simulink model "IEEE_39_case7"  (R2024b)
settings: Solver=ode3  StartTime=0  StopTime=40  FixedStep=Ts  MaxStep=1/60  RelTol=1e-3  AbsTol=1e-3  EnableMultiTasking=on
values from neighbouring files (symbols this model uses):
  c_f = c_f*Cb    [fun00_GFL_pu_2_normial.m]    (also in fun00_GFM_pu_2_normial.m)
  Dt = 0    [s02_case1.m]    (also in s02_case2.m; s03_case3.m; s03_case4.m; s03_case5.m)
  dw0_sm = 0    [s02_case1.m]    (also in s02_case2.m; s03_case3.m; s03_case4.m; s03_case5.m)
  Emax = 1.3    [s02_case1.m]    (also in s02_case2.m; s03_case3.m; s03_case4.m; s03_case5.m)
  Emin = 0.5    [s02_case1.m]    (also in s02_case2.m; s03_case3.m; s03_case4.m; s03_case5.m)
  Epss = 0.09    [s02_case1.m]    (also in s02_case2.m; s03_case3.m; s03_case4.m; s03_case5.m)
  fb = fn    (= 60)    [s02_case1.m]    (also in s02_case2.m; s03_case3.m; s03_case4.m; s03_case5.m)
  fn_sm = fn*ones(1,10)    [s02_case1.m]    (also in s02_case2.m; s03_case3.m; s03_case4.m; s03_case5.m)
  H_sm = [5,3.03,3.58,2.86,2.6,3.48,2.64,2.43,3.45,4.2]    [s02_case1.m]    (also in s02_case2.m; s03_case3.m; s03_case4.m; s03_case5.m)
  ia0_sm = 0    [s02_case1.m]    (also in s02_case2.m; s03_case3.m; s03_case4.m; s03_case5.m)
  ib0_sm = 0    [s02_case1.m]    (also in s02_case2.m; s03_case3.m; s03_case4.m; s03_case5.m)
  ic0_sm = 0    [s02_case1.m]    (also in s02_case2.m; s03_case3.m; s03_case4.m; s03_case5.m)
  Kd_sm = 0*ones(1,10)    [s02_case1.m]    (also in s02_case2.m; s03_case3.m; s03_case4.m; s03_case5.m)
  Ke = 1000    [s02_case1.m]    (also in s02_case2.m; s03_case3.m; s03_case4.m; s03_case5.m)
  ki_i = ki_i_pu*Vb_p_ph/Ib_p_ph    [fun00_GFL_pu_2_normial.m]    (also in fun00_GFM_pu_2_normial.m)
  ki_p = ki_p_pu/Sb*Ib_p_ph    [fun00_GFL_pu_2_normial.m]
  ki_pll = ki_pll/Vb_p_ph    [fun00_GFL_pu_2_normial.m]
  ki_q = ki_q_pu/Sb*Ib_p_ph    [fun00_GFL_pu_2_normial.m]
  kp_i = kp_i_pu*Vb_p_ph/Ib_p_ph    [fun00_GFL_pu_2_normial.m]    (also in fun00_GFM_pu_2_normial.m)
  kp_p = kp_p_pu/Sb*Ib_p_ph    [fun00_GFL_pu_2_normial.m]
  kp_pll = kp_pll/Vb_p_ph    [fun00_GFL_pu_2_normial.m]
  kp_q = kp_q_pu/Sb*Ib_p_ph    [fun00_GFL_pu_2_normial.m]
  Ks = 1    [s02_case1.m]    (also in s02_case2.m; s03_case3.m; s03_case4.m; s03_case5.m)
  l_f = l_f*Lb    [fun00_GFL_pu_2_normial.m]    (also in fun00_GFM_pu_2_normial.m)
  line = [     1	2	0.0035	0.0411	0.6987	0	100	345 ... (first row only)    [s02_case1.m]    (also in s02_case2.m; s03_case3.m; s03_case4.m; s03_case5.m)
  line_pu = line    [s02_case1.m]    (also in s02_case2.m; s03_case3.m; s03_case4.m; s03_case5.m)
  p = 1    [s02_case1.m]    (also in s02_case2.m; s03_case3.m; s03_case4.m; s03_case5.m)
  pha0_sm = 0    [s02_case1.m]    (also in s02_case2.m; s03_case3.m; s03_case4.m; s03_case5.m)
  phb0_sm = 0    [s02_case1.m]    (also in s02_case2.m; s03_case3.m; s03_case4.m; s03_case5.m)
  phc0_sm = 0    [s02_case1.m]    (also in s02_case2.m; s03_case3.m; s03_case4.m; s03_case5.m)
  Pn_sm = 1000*ones(1,num_gen)    [s02_case1.m]    (also in s02_case2.m; s03_case3.m; s03_case4.m; s03_case5.m)
  Pref_sm = [500 250 600 978 510 650 560 540 830 550]./Pn_sm    [s02_case1.m]    (also in s02_case2.m; s03_case3.m; s03_case4.m; s03_case5.m)
  pset = p_set_pu*Sb    [fun00_GFL_pu_2_normial.m]
  qset = q_set_pu*Sb    [fun00_GFL_pu_2_normial.m]
  R = 0.05    [s02_case1.m]    (also in s02_case2.m; s03_case3.m; s03_case4.m; s03_case5.m)
  r_f = r_f*Zb    [fun00_GFL_pu_2_normial.m]    (also in fun00_GFM_pu_2_normial.m)
  rs = 0.28    [s02_case1.m]    (also in s02_case2.m; s03_case3.m; s03_case4.m; s03_case5.m)
  Sb = 1000*10^6    (= 1000000000)    [s02_case1.m]    (also in s02_case2.m; s03_case3.m; s03_case4.m; s03_case5.m)
  T2 = 0.5    [s02_case1.m]    (also in s02_case2.m; s03_case3.m; s03_case4.m; s03_case5.m)
  T3 = 0.5    [s02_case1.m]    (also in s02_case2.m; s03_case3.m; s03_case4.m; s03_case5.m)
  t_gfl = 50    [s03_case3.m]    (also in s03_case4.m; s03_case5.m; s04_case6.m = 25; s04_case7.m = 25)
  t_gfm = 25    [s03_case3.m]    (also in s03_case4.m; s03_case5.m; s04_case6.m = 50; s04_case7.m = 50)
  t_s = 30    [s02_case1.m]    (also in s02_case2.m; s03_case3.m = 70; s03_case4.m = 70; s03_case5.m = 70)
  Te = 0.05    [s02_case1.m]    (also in s02_case2.m; s03_case3.m; s03_case4.m; s03_case5.m)
  Tfa = 3    [s02_case1.m]    (also in s02_case2.m; s03_case3.m; s03_case4.m; s03_case5.m)
  Tfb = 10    [s02_case1.m]    (also in s02_case2.m; s03_case3.m; s03_case4.m; s03_case5.m)
  theta0_sm = 0    [s02_case1.m]    (also in s02_case2.m; s03_case3.m; s03_case4.m; s03_case5.m)
  Ts = 1e-5    (= 1e-05)    [s02_case1.m]    (also in s02_case2.m; s03_case3.m; s03_case4.m; s03_case5.m)
  Ts1 = 0.76    [s02_case1.m]    (also in s02_case2.m; s03_case3.m; s03_case4.m; s03_case5.m)
  Ts2 = 0.1    [s02_case1.m]    (also in s02_case2.m; s03_case3.m; s03_case4.m; s03_case5.m)
  Ts3 = 0.76    [s02_case1.m]    (also in s02_case2.m; s03_case3.m; s03_case4.m; s03_case5.m)
  Ts4 = 0.1    [s02_case1.m]    (also in s02_case2.m; s03_case3.m; s03_case4.m; s03_case5.m)
  Ts5 = 10    [s02_case1.m]    (also in s02_case2.m; s03_case3.m; s03_case4.m; s03_case5.m)
  Un_sm = [345,22,22,22,22,22,22,22,345,22]    [s02_case1.m]    (also in s02_case2.m; s03_case3.m; s03_case4.m; s03_case5.m)
  Vb_gfm = 22*10^3    (= 22000)    [s02_case1.m]    (also in s02_case2.m; s03_case3.m; s03_case4.m; s03_case5.m)
  Vdc = 3*Vb_p_ph    [fun00_GFL_pu_2_normial.m]    (also in fun00_GFM_pu_2_normial.m)
  Vmax = 2    [s02_case1.m]    (also in s02_case2.m; s03_case3.m; s03_case4.m; s03_case5.m)
  Vmin = 0    [s02_case1.m]    (also in s02_case2.m; s03_case3.m; s03_case4.m; s03_case5.m)
  Vref_sm = 1*ones(1,10)    [s02_case1.m]    (also in s02_case2.m; s03_case3.m; s03_case4.m; s03_case5.m)
  w_b = fb*2*pi    [fun00_GFL_pu_2_normial.m]    (also in fun00_GFM_pu_2_normial.m; s02_case1.m = 376.991118431; s02_case2.m = 376.991118431; s03_case3.m = 376.991118431)
  wb = w_b    (= 376.991118431)    [s02_case1.m]    (also in s02_case2.m; s03_case3.m; s03_case4.m; s03_case5.m)
  xd = xd_t    (= 0.296)    [s02_case1.m]    (also in s02_case2.m; s03_case3.m; s03_case4.m; s03_case5.m)
undefined symbols (not defined in the file or in its folder): c_f_gfm, D1, D_p_gfm, D_p_gfm_s, D_q_gfm, Delta, DiscIntNeverNeededParam, Init, Init_GFL, J_gfm, Ka, Kf, ki_i_gfm, ki_pll_s, ki_vc_gfm, kp_i_gfm, kp_pll_s, kp_vc_gfm, l_f_gfm, P_set_gfm, Q_set_gfm, r_f_gfm, Ta, Tf, Vb, Vdc_gfm
libraries: spsThreePhaseVIMeasurementLib x76, spsabctodq0Lib x53, spsThreePhaseSeriesRLCBranchLib x52, slpidlib x50, spsThreePhaseParallelRLCLoadLib x20, spsThreePhaseTransformerTwoWindingsLib x12, spsdq0toabcLib x9, spsGroundLib x9, spsPowerPositiveSequenceLib x9, spsUniversalBridgeLib x9, spsDCVoltageSourceLib x9, spsFirstOrderFilterLib x1
(part 10 of 10)

== system IEEE_39_case7/A3/G7(GFM2)/Current Lopp ==
  Vodq : Inport
  Icdq : Inport  Port=2
  i_ref_dq : Inport  Port=3
  theta : Inport  Port=4
  Demux : Demux  Outputs=2
  Demux1 : Demux  Outputs=2
  Demux4 : Demux  Outputs=2
  Gain : Gain  Gain=2/Vdcnorm
  Mux1 : Mux  Inputs=3
  Mux3 : Mux  Inputs=2
  Mux4 : Mux  Inputs=2
  PID Controller2 : slpidlib/PID Controller  Controller=PI  Form=Parallel  TimeDomain=Continuous-time  UseExternalTs=off  SampleTime=-1  IntegratorMethod=Forward Euler  FilterMethod=Forward Euler  ControllerParametersSource=internal  P=Current_P  I=Current_I  UseKiTs=off  D=0  UseExternalDerivativeSource=off  N=100  UseFilter=on  TunerSelectOption=Transfer Function Based (PID Tuner App)  InitialConditionSource=internal  InitialConditionForIntegrator=InitialV.Vcd-InitialV.Vod  InitialConditionForFilter=0  DifferentiatorICPrevScaledInput=0  ExternalReset=none  TrackingMode=off  Kt=1  LimitOutput=off  SatLimitsSource=internal  UpperSaturationLimit=inf  LowerSaturationLimit=-inf  LinearizeAsGain=on  AntiWindupMode=none  Kb=1  LimitIntegrator=off  UpperIntegratorSaturationLimit=inf  LowerIntegratorSaturationLimit=-inf  POutMin=[]  POutMax=[]  IOutMin=[]  IOutMax=[]  DOutMin=[]  DOutMax=[]  NOutMin=[]  NOutMax=[]  SumOutMin=[]  SumOutMax=[]  SaturationOutMin=[]  SaturationOutMax=[]  PParamMin=[]  PParamMax=[]  IParamMin=[]  IParamMax=[]  DParamMin=[]  DParamMax=[]  NParamMin=[]  NParamMax=[]  KbParamMin=[]  KbParamMax=[]  KtParamMin=[]  KtParamMax=[]  KbOutMin=[]  KbOutMax=[]  KtOutMin=[]  KtOutMax=[]  IntegratorOutMin=[]  IntegratorOutMax=[]  FilterOutMin=[]  FilterOutMax=[]  SumI1OutMin=[]  SumI1OutMax=[]  SumI2OutMin=[]  SumI2OutMax=[]  SumI3OutMin=[]  SumI3OutMax=[]  SumI4OutMin=[]  SumI4OutMax=[]  SumDOutMin=[]  SumDOutMax=[]  DifferentiatorOutMin=[]  DifferentiatorOutMax=[]  FilterDiffOutCoefMin=[]  FilterDiffOutCoefMax=[]  ReciprocalOutMin=[]  ReciprocalOutMax=[]  SumDenOutMin=[]  SumDenOutMax=[]  SumNumOutMin=[]  SumNumOutMax=[]  DivideOutMin=[]  DivideOutMax=[]  UdiffTsProdOutMin=[]  UdiffTsProdOutMax=[]  NTsProdOutMin=[]  NTsProdOutMax=[]  UintegralTsProdOutMin=[]  UintegralTsProdOutMax=[]  UngainTsProdOutMin=[]  UngainTsProdOutMax=[]  ClampingZeroOutDataTypeStr=Inherit: Inherit via back propagation  ClampingZeroOutMin=[]  ClampingZeroOutMax=[]  FilterDenConstantOutDataTypeStr=Inherit: Inherit via back propagation  FilterDenConstantOutMin=[]  FilterDenConstantOutMax=[]  PCopyOutDataTypeStr=Inherit: Inherit via back propagation  PCopyOutMin=[]  PCopyOutMax=[]  NCopyOutDataTypeStr=Inherit: Inherit via back propagation  NCopyOutMin=[]  NCopyOutMax=[]  IntegratorContinuousStateAttributes=''  IntegratorStateMustResolveToSignalObject=off  IntegratorRTWStateStorageClass=Auto  FilterContinuousStateAttributes=''  FilterStateMustResolveToSignalObject=off  FilterRTWStateStorageClass=Auto  ParallelPVariant=InternalParameters  IdealPVariant=Disabled  IVariant=InternalParameters  DVariant=Disabled  IntegratorVariant=Continuous  SatVariant=Disabled  AWVariant=Passthrough  PCopyVariant=Disabled  TRVariant=Disabled  FdbkBlocksVariant=Forward  IdealPFdbkVariant=Disabled  SatFdbkVariant=Disabled  DerivativeFilterVariant=Disabled  NVariant=Disabled  NCopyVariant=Disabled_SignalSpec  FilterICVariant=Disabled  IntegratorICVariant=InternalICs  ExternalResetVariant=Disabled  TRSumVariant=Passthrough  SumFdbkVariant=Disabled  SumVariant=Sum_PI  TsampFilterVariant=InternalTs  TsampNgainVariant=Passthrough  TsampIntegralVariant=Disabled_SignalSpec  ExternalSaturationOutDataTypeStr=Inherit: Same as second input  DerivativeSourceVariant=Disabled  PreIntVariant=InternalPreInt
  PID Controller3 : slpidlib/PID Controller  Controller=PI  Form=Parallel  TimeDomain=Continuous-time  UseExternalTs=off  SampleTime=-1  IntegratorMethod=Forward Euler  FilterMethod=Forward Euler  ControllerParametersSource=internal  P=Current_P  I=Current_I  UseKiTs=off  D=0  UseExternalDerivativeSource=off  N=100  UseFilter=on  TunerSelectOption=Transfer Function Based (PID Tuner App)  InitialConditionSource=internal  InitialConditionForIntegrator=InitialV.Vcq-InitialV.Voq  InitialConditionForFilter=0  DifferentiatorICPrevScaledInput=0  ExternalReset=none  TrackingMode=off  Kt=1  LimitOutput=off  SatLimitsSource=internal  UpperSaturationLimit=inf  LowerSaturationLimit=-inf  LinearizeAsGain=on  AntiWindupMode=none  Kb=1  LimitIntegrator=off  UpperIntegratorSaturationLimit=inf  LowerIntegratorSaturationLimit=-inf  POutMin=[]  POutMax=[]  IOutMin=[]  IOutMax=[]  DOutMin=[]  DOutMax=[]  NOutMin=[]  NOutMax=[]  SumOutMin=[]  SumOutMax=[]  SaturationOutMin=[]  SaturationOutMax=[]  PParamMin=[]  PParamMax=[]  IParamMin=[]  IParamMax=[]  DParamMin=[]  DParamMax=[]  NParamMin=[]  NParamMax=[]  KbParamMin=[]  KbParamMax=[]  KtParamMin=[]  KtParamMax=[]  KbOutMin=[]  KbOutMax=[]  KtOutMin=[]  KtOutMax=[]  IntegratorOutMin=[]  IntegratorOutMax=[]  FilterOutMin=[]  FilterOutMax=[]  SumI1OutMin=[]  SumI1OutMax=[]  SumI2OutMin=[]  SumI2OutMax=[]  SumI3OutMin=[]  SumI3OutMax=[]  SumI4OutMin=[]  SumI4OutMax=[]  SumDOutMin=[]  SumDOutMax=[]  DifferentiatorOutMin=[]  DifferentiatorOutMax=[]  FilterDiffOutCoefMin=[]  FilterDiffOutCoefMax=[]  ReciprocalOutMin=[]  ReciprocalOutMax=[]  SumDenOutMin=[]  SumDenOutMax=[]  SumNumOutMin=[]  SumNumOutMax=[]  DivideOutMin=[]  DivideOutMax=[]  UdiffTsProdOutMin=[]  UdiffTsProdOutMax=[]  NTsProdOutMin=[]  NTsProdOutMax=[]  UintegralTsProdOutMin=[]  UintegralTsProdOutMax=[]  UngainTsProdOutMin=[]  UngainTsProdOutMax=[]  ClampingZeroOutDataTypeStr=Inherit: Inherit via back propagation  ClampingZeroOutMin=[]  ClampingZeroOutMax=[]  FilterDenConstantOutDataTypeStr=Inherit: Inherit via back propagation  FilterDenConstantOutMin=[]  FilterDenConstantOutMax=[]  PCopyOutDataTypeStr=Inherit: Inherit via back propagation  PCopyOutMin=[]  PCopyOutMax=[]  NCopyOutDataTypeStr=Inherit: Inherit via back propagation  NCopyOutMin=[]  NCopyOutMax=[]  IntegratorContinuousStateAttributes=''  IntegratorStateMustResolveToSignalObject=off  IntegratorRTWStateStorageClass=Auto  FilterContinuousStateAttributes=''  FilterStateMustResolveToSignalObject=off  FilterRTWStateStorageClass=Auto  ParallelPVariant=InternalParameters  IdealPVariant=Disabled  IVariant=InternalParameters  DVariant=Disabled  IntegratorVariant=Continuous  SatVariant=Disabled  AWVariant=Passthrough  PCopyVariant=Disabled  TRVariant=Disabled  FdbkBlocksVariant=Forward  IdealPFdbkVariant=Disabled  SatFdbkVariant=Disabled  DerivativeFilterVariant=Disabled  NVariant=Disabled  NCopyVariant=Disabled_SignalSpec  FilterICVariant=Disabled  IntegratorICVariant=InternalICs  ExternalResetVariant=Disabled  TRSumVariant=Passthrough  SumFdbkVariant=Disabled  SumVariant=Sum_PI  TsampFilterVariant=InternalTs  TsampNgainVariant=Passthrough  TsampIntegralVariant=Disabled_SignalSpec  ExternalSaturationOutDataTypeStr=Inherit: Same as second input  DerivativeSourceVariant=Disabled  PreIntVariant=InternalPreInt
  Scope : Scope  NumInputPorts=2
  Sum2 : Sum  Inputs=-+|
  Sum3 : Sum  Inputs=|+-
  Sum6 : Sum  Inputs=++|
  Sum7 : Sum  Inputs=|++
  Unit Delay1 : UnitDelay  SampleTime=-1  HasFrameUpgradeWarning=on
  V0 : Constant  Value=0
  VSG_ref : Scope  NumInputPorts=2
  dq0 to abc : spsdq0toabcLib/dq0 to abc  Alignment=Aligned with phase A axis
  电流对比 : Scope  NumInputPorts=2
  VSG_Uref : Outport
  wires:
  Mux4/1 -> 电流对比/1
  Mux1/1 -> Scope/1, Gain/1
  Vodq/1 -> Demux1/1
  Demux1/1 -> [Vod]
  Demux1/2 -> [Voq]
  Demux4/1 -> [Icd]
  Icdq/1 -> Demux4/1
  Demux4/2 -> [Icq]
  [Icd] -> Mux4/2
  [Icdref] -> Mux4/1
  [Icqref] -> Mux3/1
  [Icq] -> Mux3/2
  Mux3/1 -> 电流对比/2
  [Icd] -> Sum2/1
  Sum2/1 -> PID Controller2/1
  Sum3/1 -> PID Controller3/1
  V0/1 -> Mux1/3
  theta/1 -> dq0 to abc/2
  PID Controller2/1 -> Sum6/2
  PID Controller3/1 -> Sum7/1
  Sum7/1 -> Mux1/2, VSG_ref/2
  Sum6/1 -> Mux1/1, VSG_ref/1
  dq0 to abc/1 -> Unit Delay1/1
  [Icq] -> Sum3/2
  [Icdref] -> Sum2/2
  [Icqref] -> Sum3/1
  Unit Delay1/1 -> VSG_Uref/1
  Gain/1 -> dq0 to abc/1, Scope/2
  i_ref_dq/1 -> Demux/1
  Demux/1 -> [Icdref]
  Demux/2 -> [Icqref]
  [Vod] -> Sum6/1
  [Voq] -> Sum7/2

== system IEEE_39_case7/A3/G7(GFM2)/Measurement ==
  Vabc_s0 : Inport
  Iabc_s0 : Inport  Port=2
  Iabc_s2 : Inport  Port=3
  theta : Inport  Port=4
  " " : spsPowerPositiveSequenceLib/Power (Positive-Sequence)  Freq=fbnorm  Vinit=[0, 0]  Iinit=[0, 0]  Ts=0
  Add1 : Sum  Inputs=-+
  Add2 : Sum
  Demux : Demux  Outputs=2
  Demux1 : Demux  Outputs=2
  Fcn : Fcn  Expr=sqrt(u(1)^2 + u(2)^2)
  Gain : Gain
  Gain{1,3..5} (4 alike) : Gain  Gain=3/2
  Gain2 : Gain
  Mux : Mux  Inputs=2
  Mux1 : Mux  Inputs=2
  Mux2 : Mux  Inputs=2
  Product{,1..3} (4 alike) : Product
  Scope{,1..3} (4 alike) : Scope
  Selector : Selector  InputPortWidth=3  IndexOptions=Index vector (dialog)  Indices=[1 2]  OutputSizes=2
  Selector1 : Selector  InputPortWidth=3  IndexOptions=Index vector (dialog)  Indices=[1 2]  OutputSizes=2
  Selector2 : Selector  InputPortWidth=3  IndexOptions=Index vector (dialog)  Indices=[1 2]  OutputSizes=2
  True : Scope
  True P : Scope
  True Q : Scope
  abc to dq0 : spsabctodq0Lib/abc to dq0  Alignment=Aligned with phase A axis
  abc to dq3 : spsabctodq0Lib/abc to dq0  Alignment=Aligned with phase A axis
  abc to dq4 : spsabctodq0Lib/abc to dq0  Alignment=Aligned with phase A axis
  P : Outport
  Q : Outport  Port=2
  Vodq : Outport  Port=3
  Icdq : Outport  Port=4
  Vrms : Outport  Port=5
  wires:
  abc to dq0/1 -> Fcn/1, Selector/1
  theta/1 -> abc to dq4/2, abc to dq3/2, abc to dq0/2
  Add2/1 -> Mux1/2, P/1, Scope2/1
  [Voq] -> Product3/1
  Iabc_s0/1 -> " "/2, abc to dq3/1
  Iabc_s2/1 -> abc to dq4/1
  [Iod] -> Product/2
  [Vod] -> Product1/1
  Selector/1 -> Vodq/1, Demux/1, Scope/1
  [Voq] -> Product2/1
  abc to dq4/1 -> Selector2/1
  [Vod] -> Product/1
  Demux/1 -> [Vod]
  Vabc_s0/1 -> " "/1, abc to dq0/1
  Mux2/1 -> True Q/1
  Fcn/1 -> Vrms/1
  Add1/1 -> Mux2/2, Q/1, Scope3/1
  Mux1/1 -> True P/1
  Selector1/1 -> Demux1/1, Scope1/1
  abc to dq3/1 -> Selector1/1
  Product3/1 -> Gain5/1
  [Ioq] -> Product1/2
  [Iod] -> Product3/2
  Product1/1 -> Gain4/1
  Demux1/2 -> [Ioq]
  Demux1/1 -> [Iod]
  Demux/2 -> [Voq]
  Mux/1 -> True/1
  [Ioq] -> Product2/2
  Selector2/1 -> Icdq/1
  Product2/1 -> Gain3/1
  Product/1 -> Gain1/1
  " "/2 -> Gain2/1
  " "/1 -> Gain/1
  Gain/1 -> Mux1/1, Mux/1
  Gain2/1 -> Mux2/1, Mux/2
  Gain1/1 -> Add2/1
  Gain3/1 -> Add2/2
  Gain4/1 -> Add1/1
  Gain5/1 -> Add1/2

== system IEEE_39_case7/A3/G7(GFM2)/Subsystem3 ==
  theta : Inport
  Vabc : Inport  Port=2
  Iabc : Inport  Port=3
  abc to dq1 : spsabctodq0Lib/abc to dq0  Alignment=Aligned with phase A axis
  abc to dq2 : spsabctodq0Lib/abc to dq0  Alignment=Aligned with phase A axis
  Vdq0 : Outport
  Idq0 : Outport  Port=2
  wires:
  Iabc/1 -> abc to dq2/1
  theta/1 -> abc to dq2/2, abc to dq1/2
  abc to dq1/1 -> Vdq0/1
  Vabc/1 -> abc to dq1/1
  abc to dq2/1 -> Idq0/1

== system IEEE_39_case7/A3/G7(GFM2)/VSM control ==
  P : Inport
  P_set : Inport  Port=2
  Q : Inport  Port=3
  Q_set : Inport  Port=4
  Clock : Clock
  Constant : Constant  Value=2*pi*fbnorm
  Constant1 : Constant  Value=0
  Constant2 : Constant  Value=Vbnorm/sqrt(3)*sqrt(2)
  Constant3 : Constant  Value=2*pi
  Display : Display
  Gain : Gain  Gain=1/Dq
  Gain1 : Gain  Gain=Dp
  Gain2 : Gain  Gain=D_p_gfm_s(2)
  Gain6 : Gain  Gain=1/J
  Integrator : Integrator  InitialCondition=2*pi*fbnorm
  Integrator1 : Integrator
  Integrator2 : Integrator  InitialCondition=InitialV.theta0
  Mod : Math  Operator=mod
  Mux : Mux  Inputs=2
  Scope : Scope
  Sum : Sum  Inputs=-|+|-
  Sum1 : Sum  Inputs=-|+
  Sum2 : Sum  Inputs=-|+
  Sum3 : Sum  Inputs=+-|
  Switch : Switch  Threshold=t_gfm  SaturateOnIntegerOverflow=off  InputSameDT=off
  w_ref : Outport  VectorParamsAs1DForOutWhenUnconnected=off
  theta_ref : Outport  Port=2  VectorParamsAs1DForOutWhenUnconnected=off
  Vodq_ref : Outport  Port=3  VectorParamsAs1DForOutWhenUnconnected=off
  theta_output : Outport  Port=4
  theta0 : Outport  Port=5
  wires:
  [d_output] -> Sum/1
  P/1 -> Sum/3
  Gain6/1 -> Integrator/1
  P_set/1 -> Sum/2
  Sum/1 -> Gain6/1
  Sum2/1 -> [d_input], Integrator1/1
  Integrator/1 -> Sum2/2, Display/1, w_ref/1, Integrator2/1  "w"
  Constant/1 -> Sum2/1
  Q_set/1 -> Sum1/1
  Q/1 -> Sum1/2
  Sum1/1 -> Gain/1
  Constant1/1 -> Mux/2
  Mux/1 -> Vodq_ref/1
  Gain/1 -> Sum3/2
  Constant2/1 -> Sum3/1
  Sum3/1 -> Mux/1
  Integrator2/1 -> theta_output/1, Mod/1  "theta"
  Mod/1 -> theta_ref/1
  Constant3/1 -> Mod/2
  Integrator1/1 -> theta0/1, Scope/1
  Gain1/1 -> Switch/3
  [d_input] -> Gain1/1
  Clock/1 -> Switch/2
  Switch/1 -> [d_output]
  [d_input] -> Gain2/1
  Gain2/1 -> Switch/1

== system IEEE_39_case7/A3/G7(GFM2)/Voltage Loop ==
  v_ref_dq : Inport
  vo_dq : Inport  Port=2
  Demux : Demux  Outputs=2
  Demux1 : Demux  Outputs=2
  Mux : Mux  Inputs=2
  PID Controller : slpidlib/PID Controller  Controller=PI  Form=Parallel  TimeDomain=Continuous-time  UseExternalTs=off  SampleTime=-1  IntegratorMethod=Forward Euler  FilterMethod=Forward Euler  ControllerParametersSource=internal  P=Voltage_P  I=Voltage_I  UseKiTs=off  D=0  UseExternalDerivativeSource=off  N=100  UseFilter=on  TunerSelectOption=Transfer Function Based (PID Tuner App)  InitialConditionSource=internal  InitialConditionForIntegrator=InitialV.Icd  InitialConditionForFilter=0  DifferentiatorICPrevScaledInput=0  ExternalReset=none  TrackingMode=off  Kt=1  LimitOutput=off  SatLimitsSource=internal  UpperSaturationLimit=inf  LowerSaturationLimit=-inf  LinearizeAsGain=on  AntiWindupMode=none  Kb=1  LimitIntegrator=off  UpperIntegratorSaturationLimit=inf  LowerIntegratorSaturationLimit=-inf  POutMin=[]  POutMax=[]  IOutMin=[]  IOutMax=[]  DOutMin=[]  DOutMax=[]  NOutMin=[]  NOutMax=[]  SumOutMin=[]  SumOutMax=[]  SaturationOutMin=[]  SaturationOutMax=[]  PParamMin=[]  PParamMax=[]  IParamMin=[]  IParamMax=[]  DParamMin=[]  DParamMax=[]  NParamMin=[]  NParamMax=[]  KbParamMin=[]  KbParamMax=[]  KtParamMin=[]  KtParamMax=[]  KbOutMin=[]  KbOutMax=[]  KtOutMin=[]  KtOutMax=[]  IntegratorOutMin=[]  IntegratorOutMax=[]  FilterOutMin=[]  FilterOutMax=[]  SumI1OutMin=[]  SumI1OutMax=[]  SumI2OutMin=[]  SumI2OutMax=[]  SumI3OutMin=[]  SumI3OutMax=[]  SumI4OutMin=[]  SumI4OutMax=[]  SumDOutMin=[]  SumDOutMax=[]  DifferentiatorOutMin=[]  DifferentiatorOutMax=[]  FilterDiffOutCoefMin=[]  FilterDiffOutCoefMax=[]  ReciprocalOutMin=[]  ReciprocalOutMax=[]  SumDenOutMin=[]  SumDenOutMax=[]  SumNumOutMin=[]  SumNumOutMax=[]  DivideOutMin=[]  DivideOutMax=[]  UdiffTsProdOutMin=[]  UdiffTsProdOutMax=[]  NTsProdOutMin=[]  NTsProdOutMax=[]  UintegralTsProdOutMin=[]  UintegralTsProdOutMax=[]  UngainTsProdOutMin=[]  UngainTsProdOutMax=[]  ClampingZeroOutDataTypeStr=Inherit: Inherit via back propagation  ClampingZeroOutMin=[]  ClampingZeroOutMax=[]  FilterDenConstantOutDataTypeStr=Inherit: Inherit via back propagation  FilterDenConstantOutMin=[]  FilterDenConstantOutMax=[]  PCopyOutDataTypeStr=Inherit: Inherit via back propagation  PCopyOutMin=[]  PCopyOutMax=[]  NCopyOutDataTypeStr=Inherit: Inherit via back propagation  NCopyOutMin=[]  NCopyOutMax=[]  IntegratorContinuousStateAttributes=''  IntegratorStateMustResolveToSignalObject=off  IntegratorRTWStateStorageClass=Auto  FilterContinuousStateAttributes=''  FilterStateMustResolveToSignalObject=off  FilterRTWStateStorageClass=Auto  ParallelPVariant=InternalParameters  IdealPVariant=Disabled  IVariant=InternalParameters  DVariant=Disabled  IntegratorVariant=Continuous  SatVariant=Disabled  AWVariant=Passthrough  PCopyVariant=Disabled  TRVariant=Disabled  FdbkBlocksVariant=Forward  IdealPFdbkVariant=Disabled  SatFdbkVariant=Disabled  DerivativeFilterVariant=Disabled  NVariant=Disabled  NCopyVariant=Disabled_SignalSpec  FilterICVariant=Disabled  IntegratorICVariant=InternalICs  ExternalResetVariant=Disabled  TRSumVariant=Passthrough  SumFdbkVariant=Disabled  SumVariant=Sum_PI  TsampFilterVariant=InternalTs  TsampNgainVariant=Passthrough  TsampIntegralVariant=Disabled_SignalSpec  ExternalSaturationOutDataTypeStr=Inherit: Same as second input  DerivativeSourceVariant=Disabled  PreIntVariant=InternalPreInt
  PID Controller1 : slpidlib/PID Controller  Controller=PI  Form=Parallel  TimeDomain=Continuous-time  UseExternalTs=off  SampleTime=-1  IntegratorMethod=Forward Euler  FilterMethod=Forward Euler  ControllerParametersSource=internal  P=Voltage_P  I=Voltage_I  UseKiTs=off  D=0  UseExternalDerivativeSource=off  N=100  UseFilter=on  TunerSelectOption=Transfer Function Based (PID Tuner App)  InitialConditionSource=internal  InitialConditionForIntegrator=InitialV.Icq  InitialConditionForFilter=0  DifferentiatorICPrevScaledInput=0  ExternalReset=none  TrackingMode=off  Kt=1  LimitOutput=off  SatLimitsSource=internal  UpperSaturationLimit=inf  LowerSaturationLimit=-inf  LinearizeAsGain=on  AntiWindupMode=none  Kb=1  LimitIntegrator=off  UpperIntegratorSaturationLimit=inf  LowerIntegratorSaturationLimit=-inf  POutMin=[]  POutMax=[]  IOutMin=[]  IOutMax=[]  DOutMin=[]  DOutMax=[]  NOutMin=[]  NOutMax=[]  SumOutMin=[]  SumOutMax=[]  SaturationOutMin=[]  SaturationOutMax=[]  PParamMin=[]  PParamMax=[]  IParamMin=[]  IParamMax=[]  DParamMin=[]  DParamMax=[]  NParamMin=[]  NParamMax=[]  KbParamMin=[]  KbParamMax=[]  KtParamMin=[]  KtParamMax=[]  KbOutMin=[]  KbOutMax=[]  KtOutMin=[]  KtOutMax=[]  IntegratorOutMin=[]  IntegratorOutMax=[]  FilterOutMin=[]  FilterOutMax=[]  SumI1OutMin=[]  SumI1OutMax=[]  SumI2OutMin=[]  SumI2OutMax=[]  SumI3OutMin=[]  SumI3OutMax=[]  SumI4OutMin=[]  SumI4OutMax=[]  SumDOutMin=[]  SumDOutMax=[]  DifferentiatorOutMin=[]  DifferentiatorOutMax=[]  FilterDiffOutCoefMin=[]  FilterDiffOutCoefMax=[]  ReciprocalOutMin=[]  ReciprocalOutMax=[]  SumDenOutMin=[]  SumDenOutMax=[]  SumNumOutMin=[]  SumNumOutMax=[]  DivideOutMin=[]  DivideOutMax=[]  UdiffTsProdOutMin=[]  UdiffTsProdOutMax=[]  NTsProdOutMin=[]  NTsProdOutMax=[]  UintegralTsProdOutMin=[]  UintegralTsProdOutMax=[]  UngainTsProdOutMin=[]  UngainTsProdOutMax=[]  ClampingZeroOutDataTypeStr=Inherit: Inherit via back propagation  ClampingZeroOutMin=[]  ClampingZeroOutMax=[]  FilterDenConstantOutDataTypeStr=Inherit: Inherit via back propagation  FilterDenConstantOutMin=[]  FilterDenConstantOutMax=[]  PCopyOutDataTypeStr=Inherit: Inherit via back propagation  PCopyOutMin=[]  PCopyOutMax=[]  NCopyOutDataTypeStr=Inherit: Inherit via back propagation  NCopyOutMin=[]  NCopyOutMax=[]  IntegratorContinuousStateAttributes=''  IntegratorStateMustResolveToSignalObject=off  IntegratorRTWStateStorageClass=Auto  FilterContinuousStateAttributes=''  FilterStateMustResolveToSignalObject=off  FilterRTWStateStorageClass=Auto  ParallelPVariant=InternalParameters  IdealPVariant=Disabled  IVariant=InternalParameters  DVariant=Disabled  IntegratorVariant=Continuous  SatVariant=Disabled  AWVariant=Passthrough  PCopyVariant=Disabled  TRVariant=Disabled  FdbkBlocksVariant=Forward  IdealPFdbkVariant=Disabled  SatFdbkVariant=Disabled  DerivativeFilterVariant=Disabled  NVariant=Disabled  NCopyVariant=Disabled_SignalSpec  FilterICVariant=Disabled  IntegratorICVariant=InternalICs  ExternalResetVariant=Disabled  TRSumVariant=Passthrough  SumFdbkVariant=Disabled  SumVariant=Sum_PI  TsampFilterVariant=InternalTs  TsampNgainVariant=Passthrough  TsampIntegralVariant=Disabled_SignalSpec  ExternalSaturationOutDataTypeStr=Inherit: Same as second input  DerivativeSourceVariant=Disabled  PreIntVariant=InternalPreInt
  Sum : Sum  Inputs=|+-
  Sum1 : Sum  Inputs=|+-
  i_ref_dq : Outport  VectorParamsAs1DForOutWhenUnconnected=off
  wires:
  Mux/1 -> i_ref_dq/1
  v_ref_dq/1 -> Demux/1
  vo_dq/1 -> Demux1/1
  Demux/1 -> [vo_ref_d]
  Demux/2 -> [vo_ref_q]
  Demux1/1 -> [vo_d]
  Demux1/2 -> [vo_q]
  Sum/1 -> PID Controller/1
  [vo_d] -> Sum/2
  Sum1/1 -> PID Controller1/1
  [vo_q] -> Sum1/2
  PID Controller/1 -> Mux/1
  PID Controller1/1 -> Mux/2
  [vo_ref_d] -> Sum/1
  [vo_ref_q] -> Sum1/1

== system IEEE_39_case7/A3/G4/Controllers1/AVR IEEE SEXS\ST1A ==
  Vc : Inport
  Vs : Inport  Port=2
  Vref : Inport  Port=3
  AVR IEEE ST1a : Subsystem  Commented=on
  AVR SEXS : Subsystem
  Sum1 : Sum  Inputs=+-+
  Ef : Outport  VectorParamsAs1DForOutWhenUnconnected=off
  wires:
  Vc/1 -> Sum1/2
  Vref/1 -> Sum1/1
  Vs/1 -> Sum1/3
  Sum1/1 -> AVR SEXS/1(dV)
  AVR SEXS/1(Ef) -> Ef/1

== system IEEE_39_case7/A3/G4/Controllers1/Governor IEEE TGOV1 ==
  dw : Inport
  Pref : Inport  Port=2
  First-Order Filter : spsFirstOrderFilterLib/First-Order Filter  FilterType=Lowpass  Tc=T1  Ts=0  Initialize=on  Vac_Init=[0, 0, 60]  Vdc_Init=P_set  PlotResponse=off  FreqRange="[0,  200,  1]"
  Gain : Gain  Gain=1/R
  Gain1 : Gain  Gain=Dt
  Saturation : Saturate  UpperLimit=Vmax  LowerLimit=Vmin
  Sum : Sum  Inputs=|+-
  Sum1 : Sum  Inputs=|+-
  Transfer Fcn1 : TransferFcn  Numerator=[T2 1]  Denominator=[T3 1]
  Pm : Outport  VectorParamsAs1DForOutWhenUnconnected=off
  wires:
  First-Order Filter/1 -> Saturation/1
  Sum1/1 -> First-Order Filter/1
  Gain1/1 -> Sum/2
  Saturation/1 -> Transfer Fcn1/1
  Sum/1 -> Pm/1
  Transfer Fcn1/1 -> Sum/1
  Gain/1 -> Sum1/2
  Pref/1 -> Sum1/1
  dw/1 -> Gain1/1, Gain/1

== system IEEE_39_case7/A3/G4/Controllers1/Measures ==
  Ua : Inport
  Ub : Inport  Port=2
  Uc : Inport  Port=3
  omega : Inport  Port=4
  Constant : Constant  Value=2*pi
  Demux : Demux  Outputs=3
  Gain : Gain  Gain=wb
  Integrator : Integrator
  Mod : Math  Operator=mod
  Mux : Mux  Inputs=3
  Product3 : Product
  Product4 : Product
  Sqrt1 : Sqrt
  Sum1 : Sum
  Terminator : Terminator
  abc to dq0 : spsabctodq0Lib/abc to dq0  Alignment=90 degrees behind phase A axis
  Uabs : Outport
  wires:
  Integrator/1 -> Gain/1
  Sqrt1/1 -> Uabs/1
  Product3/1 -> Sum1/1
  Mux/1 -> abc to dq0/1
  Demux/2 -> Product4/2, Product4/1
  Product4/1 -> Sum1/2
  Sum1/1 -> Sqrt1/1
  abc to dq0/1 -> Demux/1
  Demux/1 -> Product3/1, Product3/2
  Uc/1 -> Mux/3
  omega/1 -> Integrator/1
  Ua/1 -> Mux/1
  Ub/1 -> Mux/2
  Mod/1 -> abc to dq0/2
  Gain/1 -> Mod/1
  Constant/1 -> Mod/2
  Demux/3 -> Terminator/1

== system IEEE_39_case7/A3/G4/Controllers1/PSS IEEE PSS1A ==
  dP : Inport
  Gain : Gain  Gain=Ks
  Saturation : Saturate  UpperLimit=Epss  LowerLimit=-Epss  ZeroCross=off
  Transfer Fcn : TransferFcn  Numerator=[Ts1 1]  Denominator=[Ts2 1]
  Transfer Fcn1 : TransferFcn  Numerator=[Ts5 0]  Denominator=[Ts5 1]
  Transfer Fcn2 : TransferFcn  Numerator=[Ts3 1]  Denominator=[Ts4 1]
  Vs : Outport  VectorParamsAs1DForOutWhenUnconnected=off
  wires:
  Transfer Fcn/1 -> Transfer Fcn2/1
  Gain/1 -> Transfer Fcn1/1
  dP/1 -> Transfer Fcn/1
  Transfer Fcn2/1 -> Gain/1
  Transfer Fcn1/1 -> Saturation/1
  Saturation/1 -> Vs/1

== system IEEE_39_case7/A3/G4/Controllers1/AVR IEEE SEXS\ST1A/AVR IEEE ST1a ==
  dV : Inport
  Sum : Sum  Inputs=|+-
  Transfer Fcn1 : TransferFcn  Numerator=[Ka]  Denominator=[Ta 1]
  Transfer Fcn2 : TransferFcn  Numerator=[Kf 0]  Denominator=[Tf 1]
  Ef : Outport  VectorParamsAs1DForOutWhenUnconnected=off
  wires:
  Transfer Fcn1/1 -> Transfer Fcn2/1, Ef/1
  Sum/1 -> Transfer Fcn1/1
  dV/1 -> Sum/1
  Transfer Fcn2/1 -> Sum/2

== system IEEE_39_case7/A3/G4/Controllers1/AVR IEEE SEXS\ST1A/AVR SEXS ==
  dV : Inport
  Saturation : Saturate  UpperLimit=Emax  LowerLimit=Emin  ZeroCross=off
  Transfer Fcn : TransferFcn  Numerator=[Tfa 1]  Denominator=[Tfb 1]
  Transfer Fcn1 : TransferFcn  Numerator=[Ke]  Denominator=[Te 1]
  Ef : Outport  VectorParamsAs1DForOutWhenUnconnected=off
  wires:
  Saturation/1 -> Ef/1
  Transfer Fcn1/1 -> Saturation/1
  Transfer Fcn/1 -> Transfer Fcn1/1
  dV/1 -> Transfer Fcn/1
